simulink model "Utkarsh_2005574_W1_P5"  (R2020b)
settings: Solver=VariableStepAuto  StartTime=0.0  StopTime=10.0  RelTol=1e-3
PostLoadFcn:
  | R=10;
  | C=0.00001;
InitFcn:
  | R=10;
  | C=0.00001;
settings Model: Creator=home  LastModifiedBy=home

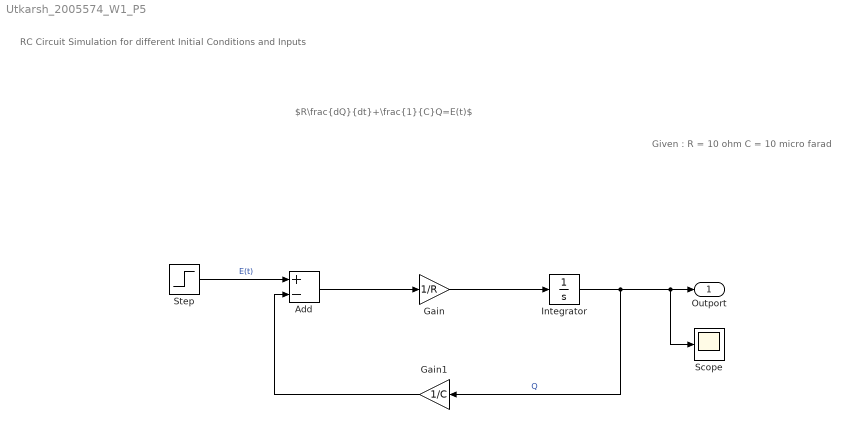
== system Utkarsh_2005574_W1_P5 ==
  note: $R\frac{dQ}{dt}+\frac{1}{C}Q=E(t)$
  note: Given :
      | R = 10 ohm
      | C = 10 micro farad
  note: RC Circuit Simulation for different Initial Conditions and Inputs
  Add : Sum  Inputs=+-
  Gain : Gain  Gain=1/R
  Gain1 : Gain  Gain=1/C
  Integrator : Integrator
  Scope : Scope
  Step : Step  SampleTime=0
  Outport : Outport
  wires:
  Step/1 -> Add/1  "E(t)"
  Add/1 -> Gain/1
  Gain/1 -> Integrator/1
  Integrator/1 -> Gain1/1, Scope/1, Outport/1  "Q"
  Gain1/1 -> Add/2
